simulink model "compilation_2_sc_user_interface"  (Simulink 7.8)
settings: Solver=ode4  SolverMode=SingleTasking  StartTime=0.0  StopTime=inf  FixedStep=0.001  RelTol=1e-3
libraries: opal_lib x3, simulink x1
Description:
  | Model of a simple control system for use iin training.
settings Model: Creator=Paul Baracos  LastModifiedBy=emma
settings DataIOCC: SaveOutput=off  SaveTime=off  SignalLoggingName=sigsOut
settings OptimizationCC: BlockReduction=off  BooleanDataType=off  InlineInvariantSignals=on  InitFltsAndDblsToZero=on
settings DebuggingCC: SaveWithParameterizedLinksMsg=none  SignalResolutionControl=TryResolveAllWithWarning  SolverPrmCheckMsg=none  MultiTaskDSMMsg=warning  MultiTaskCondExecSysMsg=none  FcnCallInpInsideContextMsg=Use local settings  StrictBusMsg=None
settings HardwareCC: TargetUnknown=on
settings RTWCC: GenCodeOnly=on  IncludeERTFirstTime=on
settings GRTTargetCC: TargetFcnLib=ansi_tfl_tmw.mat

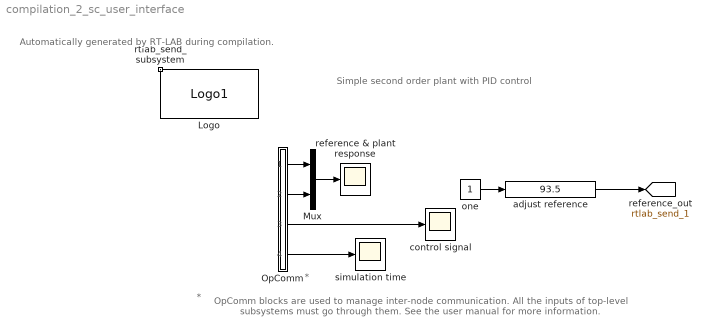
== system compilation_2_sc_user_interface ==
  note: *
  note: *
  note: OpComm blocks are used to manage inter-node communication. All the inputs of top-level
      | subsystems must go through them. See the user manual for more information.
  note: Simple second order plant with PID control
  note: Automatically generated by RT-LAB during compilation.
  Logo : opal_lib/Logo1  vide=[]
  Mux : Mux  Inputs=2
  OpComm : Subsystem
      mask init:
      | opmaskdisplay('maskdisplay_block',gcb,'disp(''OpComm'')');
      mask Display:
      | patch([0 0.5 0.7 0],[1 1 0 0],[0.7 0.75 0.9]);
      | patch([1 0.53 0.73 1],[1 1 0 0],[1 0.8 0.7]);
      | plot([0 0 1 1 0],[0 1 1 0 0]);
      | disp('OpComm')
  adjust reference : simulink/Math Operations/Slider Gain  low=0  gain=93.5  high=100
  control signal : Scope
      settings: YMin=-200  YMax=200  SaveName=controlSignal
  one : Constant
  reference & plant response : Scope
      settings: Tag=op_tm_save_it  TimeRange=10  YMin=0  YMax=160  SaveName=referenceAndPlant
  rtlab_send_subsystem : Subsystem  Priority=-100
      mask Display: text(0,0,'');
  simulation time : Scope
      settings: YMin=-200  YMax=200  SaveName=controlSignal1
  tag scope: rtlab_send_1=global
  wires:
  OpComm/4(Out4) -> simulation time/1
  one/1 -> adjust reference/1
  adjust reference/1 -> [rtlab_send_1]
  OpComm/3(Out3) -> control signal/1
  OpComm/2(Out2) -> Mux/2
  OpComm/1(Out1) -> Mux/1
  Mux/1 -> reference & plant response/1

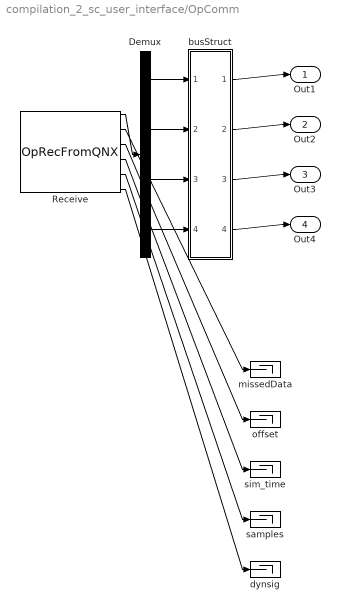
== system compilation_2_sc_user_interface/OpComm ==
  Demux : Demux  Outputs="[1  1  1  1]"
  Receive : opal_lib/Communication/OpRecFromQNX  Node_num=1  Acqu_Group=1  Data_Width=4  Synchronization=on  Interpolation=on  Threshold=1.0  modelname=compilation.mdl  sampletime=0.001
  busStruct : Subsystem
  dynsig : Terminator
  missedData : Terminator
  offset : Terminator
  samples : Terminator
  sim_time : Terminator
  Out1 : Outport
  Out2 : Outport  Port=2
  Out3 : Outport  Port=3
  Out4 : Outport  Port=4
  wires:
  Demux/4 -> busStruct/4(In4)
  Demux/3 -> busStruct/3(In3)
  Demux/2 -> busStruct/2(In2)
  Demux/1 -> busStruct/1(In1)
  busStruct/4(Out4) -> Out4/1
  busStruct/3(Out3) -> Out3/1
  busStruct/2(Out2) -> Out2/1
  busStruct/1(Out1) -> Out1/1
  Receive/1 -> Demux/1
  Receive/6 -> dynsig/1
  Receive/5 -> samples/1
  Receive/4 -> sim_time/1
  Receive/3 -> offset/1
  Receive/2 -> missedData/1

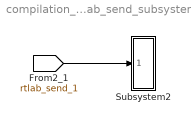
== system compilation_2_sc_user_interface/rtlab_send_subsystem ==
  Subsystem2 : Subsystem
  wires:
  [rtlab_send_1] -> Subsystem2/1(In1)

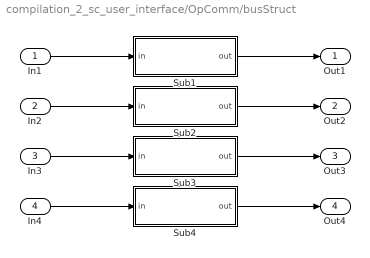
== system compilation_2_sc_user_interface/OpComm/busStruct ==
  In1 : Inport
  In2 : Inport  Port=2
  In3 : Inport  Port=3
  In4 : Inport  Port=4
  Sub1 : Subsystem
  Sub2 : Subsystem
  Sub3 : Subsystem
  Sub4 : Subsystem
  Out1 : Outport
  Out2 : Outport  Port=2
  Out3 : Outport  Port=3
  Out4 : Outport  Port=4
  wires:
  Sub4/1(out) -> Out4/1
  In4/1 -> Sub4/1(in)
  Sub3/1(out) -> Out3/1
  In3/1 -> Sub3/1(in)
  Sub2/1(out) -> Out2/1
  In2/1 -> Sub2/1(in)
  Sub1/1(out) -> Out1/1
  In1/1 -> Sub1/1(in)

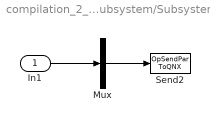
== system compilation_2_sc_user_interface/rtlab_send_subsystem/Subsystem2 ==
  In1 : Inport  PortDimensions=1
  Mux : Mux  Inputs=1
  Send2 : opal_lib/Communication/OpSendPar ToQNX  Node_num=1  modelname=compilation
  wires:
  Mux/1 -> Send2/1
  In1/1 -> Mux/1

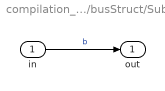
== system compilation_2_sc_user_interface/OpComm/busStruct/Sub1 ==
  in : Inport
  out : Outport
  wires:
  in/1 -> out/1  "b"

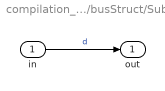
== system compilation_2_sc_user_interface/OpComm/busStruct/Sub2 ==
  in : Inport
  out : Outport
  wires:
  in/1 -> out/1  "d"

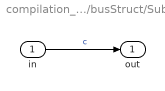
== system compilation_2_sc_user_interface/OpComm/busStruct/Sub3 ==
  in : Inport
  out : Outport
  wires:
  in/1 -> out/1  "c"

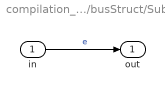
== system compilation_2_sc_user_interface/OpComm/busStruct/Sub4 ==
  in : Inport
  out : Outport
  wires:
  in/1 -> out/1  "e"
